simulink model "wamjc7"  (Simulink 8.3)
settings: Solver=ode4  SolverMode=SingleTasking  StartTime=0.0  StopTime=inf  FixedStep=sample_time  RelTol=1e-3
values from neighbouring files (symbols this model uses):
  arm_home = [ -0.1106   -1.9490   -0.1920    3.1840 ]    [NEW_PID_4DOF.m]    (also in SetPoint_Control.m = [ -0.1106   -1.9490   -0.1920    3.1840    0.2825    0.0969 ; Stochastic_coriolis.m = [  -0.1106   -1.9490   -0.1920    3.1840    0.2825    0.0969; Untitled4.m = [ -0.1106   -1.9490   -0.1920    3.1840    0.2825    0.0969 )
  b = 0.001    [DC_motor.m]    (also in SetPoint_Control.m = diag(100*ones(7,1)))
  C = Cjk(q)    [B.m]    (also in DC_motor.m = [1  0  0]; ILC_Grav_Comp.m = [zeros(7,7),eye(7)]; ILC_Grav_Comp_Diff.m = [zeros(7,7),eye(7)]; ILC_Grav_comp_Kalman.m = [zeros(7,7),eye(7)])
undefined symbols (not defined in the file or in its folder): arm_home_norest, arm_j2mt, arm_m2jp, bit, CAN_init, enc_per_rev, FT_init, hand_on, MT_init, puck_I_per_Nm, rotFT2Hand, sample_time, Standard, VL1_init, VL2_init
libraries: xpclib x43, simulink x27, xpcutilitieslib x6, dspmathops x1, dspadpt3 x1, dspindex x1, dspbuff3 x1
(part 1 of 5)
settings Model: xpc_rtwmakecfg_data=_xpccanac2pci_  Creator=Matt Courtney  LastModifiedBy=paulghanem  BufferReuse=off
settings OptimizationCC: BlockReduction=off  BooleanDataType=off  OptimizeBlockIOStorage=off  BufferReuse=off  GlobalBufferReuse=off  ExpressionFolding=off  ExpressionDepthLimit=2147483647  LocalBlockOutputs=off  InitFltsAndDblsToZero=on
settings DebuggingCC: FcnCallInpInsideContextMsg=UseLocalSettings  StrictBusMsg=Warning
settings HardwareCC: ProdIntDivRoundTo=Zero  ProdEndianess=LittleEndian  ProdHWDeviceType=Generic->32-bit x86 compatible
settings SFSimCC: SimParseCustomCode=off
settings RTWCC: SystemTargetFile=xpctarget.tlc  TemplateMakefile=xpc_default_tmf  Description=xPC Target  ProcessScript=xpctarget_make_rtw_hook  RTWCompilerOptimization=On
settings TargetCC: CodeReplacementLibrary=XPC_BLAS  ParMdlRefBuildCompliant=on  ConcurrentExecutionCompliant=on  MatFileLogging=on  EnableShiftOperators=on
settings CustomProperty: DataType=string  Value=Real-Time

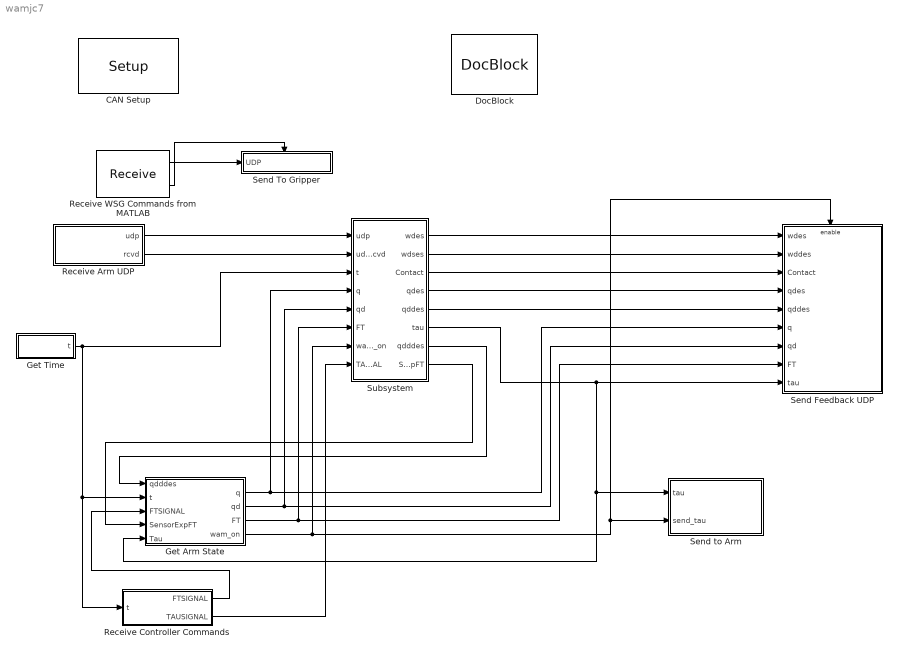
== system wamjc7 ==
  "CAN Setup " : xpclib/CAN/Softing/CAN-AC2-PCI SJA 1000/Setup   board=1  can1bus=Highspeed (ISO 11898)  can1Baudrate=1 MBaud  can1UserBR=[1,1,4,3]  can2bus=Highspeed (ISO 11898)  can2Baudrate=1 MBaud  can2UserBR=[1,1,4,3]  init=[VL1_init,VL2_init,CAN_init,MT_init,FT_init]  term=[]  bus_off_out=off  bus_off_rec=Off  ioBaseAddress=-1
  DocBlock : simulink/Model-Wide Utilities/DocBlock  DocumentType=Text
      content=|
      | This model is a very powerful controller for controlling both the Barrett
      | arm and hand at the same time and in a coordinated fashion. The uppermost
      | block you are looking at contains some CAN initialization commands, as well
      | as the closed loop controllers for the arm and hand. The hand controller
      | is fed the current arm position and velocity every cycle so that it can
      | use this information to intelligently update grasps. Double click the
      | blocks to look at more of the details of each subsystem.
  Get Arm State : Subsystem
  Get Time : Subsystem
  Receive Arm UDP : Subsystem
  Receive Controller Commands : Subsystem
  Receive WSG Commands from MATLAB : xpclib/UDP/Receive  ipAddress=192.168.1.11  ipPort=1500  width=266  vblLen=on  sampletime=sample_time
  Send Feedback UDP : Subsystem
  Send To Gripper : Subsystem  TreatAsAtomicUnit=on
  Send to Arm : Subsystem
  Subsystem : Subsystem
  wires:
  Subsystem/6(tau) -> Send Feedback UDP/9(tau), Send to Arm/1(tau), Get Arm State/5(Tau)
  Get Arm State/1(q) -> Send Feedback UDP/6(q), Subsystem/4(q)
  Get Time/1(t) -> Get Arm State/2(t), Receive Controller Commands/1(t), Subsystem/3(t)
  Subsystem/2(wdses) -> Send Feedback UDP/2(wddes)
  Subsystem/1(wdes) -> Send Feedback UDP/1(wdes)
  Receive Arm UDP/1(udp) -> Subsystem/1(udp)
  Receive Arm UDP/2(rcvd) -> Subsystem/2(udp_rcvd)
  Get Arm State/3(FT) -> Send Feedback UDP/8(FT), Subsystem/6(FT)
  Get Arm State/4(wam_on) -> Send to Arm/2(send_tau), Send Feedback UDP/Enable, Subsystem/7(wam_on)
  Get Arm State/2(qd) -> Send Feedback UDP/7(qd), Subsystem/5(qd)
  Receive Controller Commands/1(FTSIGNAL) -> Get Arm State/3(FTSIGNAL)
  Receive WSG Commands from MATLAB/1 -> Send To Gripper/1(UDP)
  Receive WSG Commands from MATLAB/2 -> Send To Gripper/Trigger
  Subsystem/4(qdes) -> Send Feedback UDP/4(qdes)
  Subsystem/5(qddes) -> Send Feedback UDP/5(qddes)
  Subsystem/7(qdddes) -> Get Arm State/1(qdddes)
  Subsystem/8(SensorExpFT) -> Get Arm State/4(SensorExpFT)
  Subsystem/3(Contact) -> Send Feedback UDP/3(Contact)
  Receive Controller Commands/2(TAUSIGNAL) -> Subsystem/8(TAUSIGNAL)

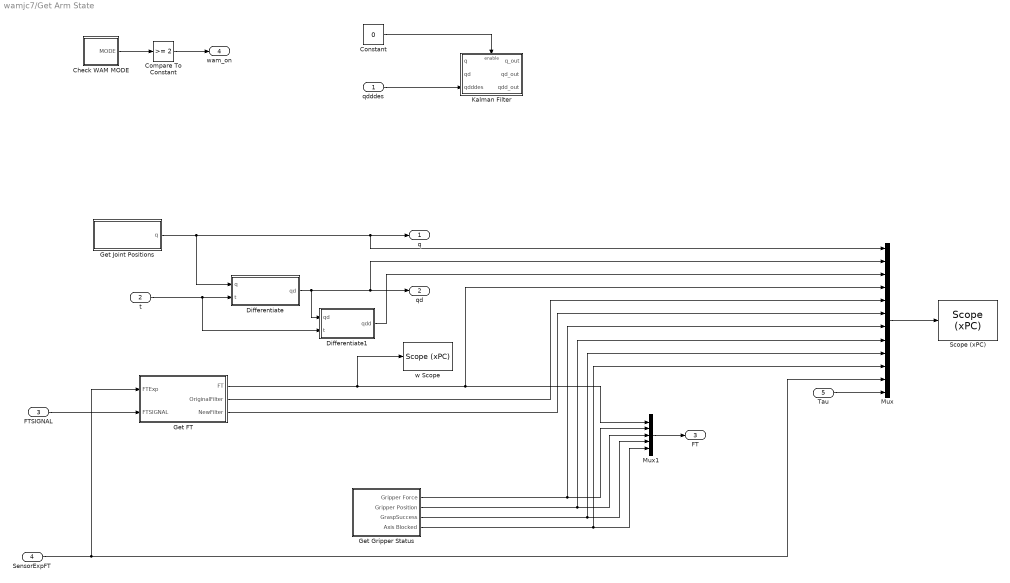
== system wamjc7/Get Arm State ==
  qdddes : Inport
  t : Inport  Port=2
  FTSIGNAL : Inport  Port=3
  SensorExpFT : Inport  Port=4
  Tau : Inport  Port=5
  Check WAM MODE : Subsystem
  Compare To Constant : simulink/Logic and Bit Operations/Compare To Constant  relop=>=  const=2  OutDataTypeStr=uint8  ZeroCross=off
  Constant : Constant  Value=0
  Differentiate : Subsystem
  Differentiate1 : Subsystem
  Get FT : Subsystem
  Get Gripper Status : Subsystem
  Get Joint Positions : Subsystem
  Kalman Filter : Subsystem
  Mux : Mux  Inputs=[7 7 7 6 6 6 1 1 1 1 6 7]
  Mux1 : Mux  Inputs=[6 1 1 1 1]
  "Scope (xPC) " : xpclib/Misc./Scope (xPC)   scopeno=3  scopetype=File  autostart=on  viewmode=Graphical redraw  formatstr='%15.6f'  grid=on  ylimits=[0,0]  nosamples=250  noprepostsamples=0  interleave=1  triggermode=FreeRun  triggersignal=1  triggerlevel=0.0  triggerslope=Either  triggerscope=1  triggersample=0  filename=QFT<%%%>.dat  mode=Lazy  writesize=512  autorestart=on  dynamicfilemode=on  maxwritefilesize=512*1024^2
  w Scope : xpclib/Misc./Scope (xPC)   scopeno=5  scopetype=Target  autostart=on  viewmode=Numerical  formatstr=['Fx %10.5f,Fy %10.5f,Fz %10.5f,TauX %10.5f,TauY %10.5f,TauZ%10.5f']  grid=on  ylimits=[0,0]  nosamples=1/(10*sample_time)  noprepostsamples=0  interleave=1  triggermode=FreeRun  triggersignal=1  triggerlevel=0.0  triggerslope=Either  triggerscope=1  triggersample=0  filename=data.dat  mode=Lazy  writesize=512  autorestart=off  dynamicfilemode=off  maxwritefilesize=512*1024^2
  q : Outport
  qd : Outport  Port=2
  FT : Outport  Port=3
  wam_on : Outport  Port=4
  wires:
  Check WAM MODE/1(MODE) -> Compare To Constant/1
  Differentiate/1(qd) -> Differentiate1/1(qd), qd/1, Mux/2
  Compare To Constant/1 -> wam_on/1
  t/1 -> Differentiate/2(t), Differentiate1/2(t)
  Get Joint Positions/1(q) -> q/1, Mux/1, Differentiate/1(q)
  Mux/1 -> "Scope (xPC) "/1
  Get FT/1(FT) -> w Scope/1, Mux/4, Mux1/1
  FTSIGNAL/1 -> Get FT/2(FTSIGNAL)
  Get FT/2(OriginalFilter) -> Mux/5
  Get FT/3(NewFilter) -> Mux/6
  Differentiate1/1(qdd) -> Mux/3
  Get Gripper Status/1(Gripper Force) -> Mux1/2, Mux/7
  Mux1/1 -> FT/1
  Get Gripper Status/2(Gripper Position) -> Mux1/3, Mux/8
  Get Gripper Status/3(GraspSuccess) -> Mux1/4, Mux/9
  Get Gripper Status/4(Axis Blocked) -> Mux1/5, Mux/10
  Tau/1 -> Mux/12
  Constant/1 -> Kalman Filter/Enable
  qdddes/1 -> Kalman Filter/3(qdddes)
  SensorExpFT/1 -> Get FT/1(FTExp), Mux/11

== system wamjc7/Get Time ==
  Clock Frequency : Constant  Value=1.193e6
  Divide1 : Product  Inputs=*/
  "xPC Target  Time " : xpclib/Misc./xPC Target  Time   ts=sample_time
  t : Outport
  wires:
  "xPC Target  Time "/1 -> Divide1/1
  Clock Frequency/1 -> Divide1/2
  Divide1/1 -> t/1

== system wamjc7/Receive Arm UDP ==
  DocBlock : simulink/Model-Wide Utilities/DocBlock  DocumentType=Text
      content=|
      | We receive UDP trajectory points on port 20202 (for arm). Right now even
      | the gains are sending over UDP but once we find some good gains they should
      | be hard coded in and should not come over UDP. The memory block and logical
      | OR at the bottom is used to check whether or not we have received data
      | since the model started running. If so, we should pass along that data,
      | otherwise we should pass the current position (i.e. the same as being in
      | gravity compensation until some UDP is received)
  Receive : xpclib/UDP/Receive  ipAddress=192.168.1.11  ipPort=5555  width=5992  vblLen=off  sampletime=sample_time
  Unpack : xpclib/UDP/Unpack  dimensions={[749,1]}  datatypes={'double'}  byteAlign=1
  udp : Outport
  rcvd : Outport  Port=2
  wires:
  Unpack/1 -> udp/1
  Receive/1 -> Unpack/1
  Receive/2 -> rcvd/1

== system wamjc7/Receive Controller Commands ==
  t : Inport
  Detect Rise Positive : simulink/Logic and Bit Operations/Detect Rise Positive  vinit=0  InputProcessing=Inherited  OutDataTypeStr=uint8
  DocBlock : simulink/Model-Wide Utilities/DocBlock  DocumentType=Text
  Embedded MATLAB Function : MATLAB Function  TreatAsAtomicUnit=on
  Receive : xpclib/UDP/Receive  ipAddress=192.168.1.11  ipPort=6666  width=9  vblLen=off  sampletime=sample_time
  Unpack : xpclib/UDP/Unpack  dimensions={[9,1]}  datatypes={'uint8'}  byteAlign=1
  FTSIGNAL : Outport
  TAUSIGNAL : Outport  Port=2
  wires:
  Receive/1 -> Unpack/1
  Receive/2 -> Detect Rise Positive/1
  Detect Rise Positive/1 -> Embedded MATLAB Function/3(rcvd)
  Unpack/1 -> Embedded MATLAB Function/2(data)
  t/1 -> Embedded MATLAB Function/1(t)
  Embedded MATLAB Function/1(FTSIGNAL) -> FTSIGNAL/1
  Embedded MATLAB Function/2(TAUSIGNAL) -> TAUSIGNAL/1

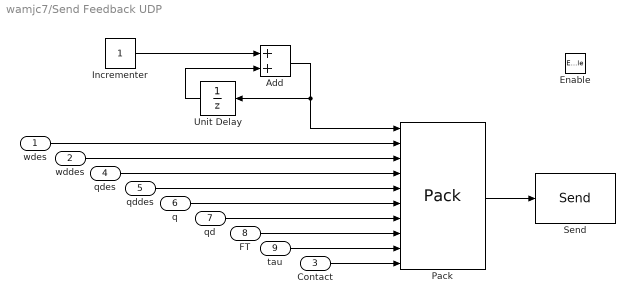
== system wamjc7/Send Feedback UDP ==
  wdes : Inport
  wddes : Inport  Port=2
  Contact : Inport  Port=3
  qdes : Inport  Port=4
  qddes : Inport  Port=5
  q : Inport  Port=6
  qd : Inport  Port=7
  FT : Inport  Port=8
  tau : Inport  Port=9
  Enable : EnablePort  PropagateVarSize=During execution
  Add : Sum  OutDataTypeStr=uint32
  Incrementer : Constant  OutDataTypeStr=uint32
  Pack : xpclib/UDP/Pack  datatypes={'uint32','double','double','double','double','double','double','double','double','double'}  byteAlign=1
  Send : xpclib/UDP/Send  ipAddress=192.168.1.11  ipPort=3333  localPort=-1  vblLen=off  sampletime=sample_time
  Unit Delay : UnitDelay  SampleTime=-1
  wires:
  Pack/1 -> Send/1
  Incrementer/1 -> Add/1
  Unit Delay/1 -> Add/2
  Add/1 -> Pack/1, Unit Delay/1
  qd/1 -> Pack/7
  q/1 -> Pack/6
  qddes/1 -> Pack/5
  qdes/1 -> Pack/4
  wddes/1 -> Pack/3
  wdes/1 -> Pack/2
  tau/1 -> Pack/9
  FT/1 -> Pack/8
  Contact/1 -> Pack/10

== system wamjc7/Send To Gripper ==
  UDP : Inport
  Trigger : TriggerPort
  Send to Gripper : xpclib/UDP/Send  ipAddress=192.168.1.20  ipPort=1500  localPort=-1  vblLen=off  sampletime=-1
  wires:
  UDP/1 -> Send to Gripper/1

== system wamjc7/Send to Arm ==
  tau : Inport
  send_tau : Inport  Port=2
  DocBlock : simulink/Model-Wide Utilities/DocBlock  DocumentType=Text
  Joint Torque to Motor Current : Subsystem
  Pack and Send Torque Packets : Subsystem
  Switch : Switch  Criteria=u2 ~= 0  Threshold=2
  Zero Torques : Constant  Value=[ 0 0 0 0 0 0 0]'  OutDataTypeStr=double
  wires:
  Joint Torque to Motor Current/1(iM) -> Pack and Send Torque Packets/1(Current)
  tau/1 -> Switch/1
  Zero Torques/1 -> Switch/3
  Switch/1 -> Joint Torque to Motor Current/1(tauJ)
  send_tau/1 -> Switch/2

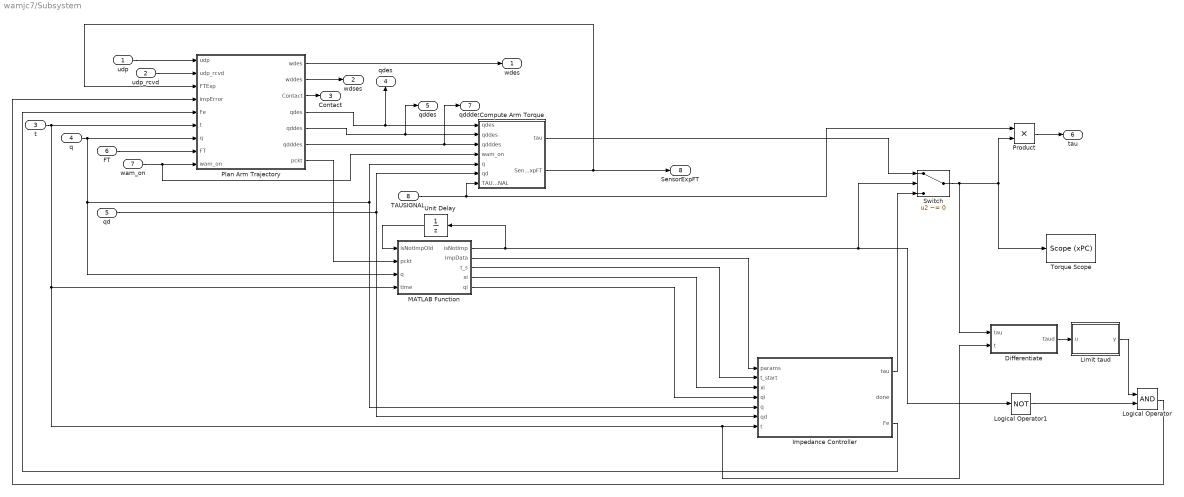
== system wamjc7/Subsystem ==
  udp : Inport
  udp_rcvd : Inport  Port=2
  t : Inport  Port=3
  q : Inport  Port=4
  qd : Inport  Port=5
  FT : Inport  Port=6
  wam_on : Inport  Port=7
  TAUSIGNAL : Inport  Port=8
  Compute Arm Torque : Subsystem
  Differentiate : Subsystem
  Impedance Controller : Subsystem
  Limit taud : MATLAB Function  TreatAsAtomicUnit=on
  Logical Operator : Logic  AllPortsSameDT=off  OutDataTypeStr=boolean
  Logical Operator1 : Logic  Operator=NOT  AllPortsSameDT=off  OutDataTypeStr=boolean
  MATLAB Function : MATLAB Function  TreatAsAtomicUnit=on
  Plan Arm Trajectory : Subsystem
  Product : Product  RndMeth=Zero
  Switch : Switch  Criteria=u2 ~= 0
  Torque Scope : xpclib/Misc./Scope (xPC)   scopeno=10  scopetype=Target  autostart=on  viewmode=Numerical  formatstr=['joint_1 %10.5f N-m,joint_2 %10.5f N-m,joint_3 %10.5f N-m,joint_4 %10.5f N-m,joint_5 %10.5f N-m,joint_6 %10.5f N-m,joint_7 %10.5f N-m']  grid=on  ylimits=[0,0]  nosamples=1/(10*sample_time)  noprepostsamples=0  interleave=1  triggermode=FreeRun  triggersignal=1  triggerlevel=0.0  triggerslope=Either  triggerscope=1  triggersample=0  filename=data.dat  mode=Lazy  writesize=512  autorestart=off  dynamicfilemode=off  maxwritefilesize=512*1024^2
  Unit Delay : UnitDelay  SampleTime=-1
  wdes : Outport
  wdses : Outport  Port=2
  Contact : Outport  Port=3
  qdes : Outport  Port=4
  qddes : Outport  Port=5
  tau : Outport  Port=6
  qdddes : Outport  Port=7
  SensorExpFT : Outport  Port=8
  wires:
  Plan Arm Trajectory/5(qddes) -> qddes/1, Compute Arm Torque/2(qddes)
  Plan Arm Trajectory/6(qdddes) -> Compute Arm Torque/3(qdddes), qdddes/1
  Compute Arm Torque/2(SensorExpFT) -> SensorExpFT/1, Plan Arm Trajectory/3(FTExp)
  t/1 -> Plan Arm Trajectory/6(t), MATLAB Function/4(time), Impedance Controller/7(t), Differentiate/2(t)
  qd/1 -> Compute Arm Torque/6(qd), Impedance Controller/6(qd)
  wam_on/1 -> Plan Arm Trajectory/9(wam_on), Compute Arm Torque/4(wam_on)
  Plan Arm Trajectory/1(wdes) -> wdes/1
  udp/1 -> Plan Arm Trajectory/1(udp)
  udp_rcvd/1 -> Plan Arm Trajectory/2(udp_rcvd)
  Plan Arm Trajectory/2(wddes) -> wdses/1
  Plan Arm Trajectory/3(Contact) -> Contact/1
  FT/1 -> Plan Arm Trajectory/8(FT)
  Unit Delay/1 -> MATLAB Function/1(isNotImpOld)
  MATLAB Function/1(isNotImp) -> Unit Delay/1, Switch/2, Logical Operator1/1
  Plan Arm Trajectory/7(pckt) -> MATLAB Function/2(pckt)
  MATLAB Function/2(ImpData) -> Impedance Controller/1(params)
  MATLAB Function/3(t_s) -> Impedance Controller/2(t_start)
  Impedance Controller/1(tau) -> Switch/3
  Compute Arm Torque/1(tau) -> Switch/1
  Switch/1 -> Differentiate/1(tau), Product/2, Torque Scope/1
  Plan Arm Trajectory/4(qdes) -> Compute Arm Torque/1(qdes), qdes/1
  MATLAB Function/4(xi) -> Impedance Controller/3(xi)
  MATLAB Function/5(qi) -> Impedance Controller/4(qi)
  Differentiate/1(taud) -> Limit taud/1(u)
  Limit taud/1(y) -> Logical Operator/1
  Logical Operator1/1 -> Logical Operator/2
  Logical Operator/1 -> Plan Arm Trajectory/4(impError)
  Impedance Controller/3(Fe) -> Plan Arm Trajectory/5(Fe)
  q/1 -> Plan Arm Trajectory/7(q), MATLAB Function/3(q), Compute Arm Torque/5(q), Impedance Controller/5(q)
  TAUSIGNAL/1 -> Compute Arm Torque/7(TAUSIGNAL), Product/1
  Product/1 -> tau/1

== system wamjc7/Get Arm State/Check WAM MODE ==
  note: Send to lower arm
  "Bit Packing " : xpcutilitieslib/Bit Packing   MaskBitPatterns={[0:7]}  MaskPackDataType=double  MaskPackDataSize=[1]
  Bit Unpacking : xpclib/CAN/Utilities/CAN bit-unpacking   bitpatterns={[16:31]}  dtypes={ 'int16'}
  DocBlock : simulink/Model-Wide Utilities/DocBlock  DocumentType=Text
      content=|
      | Here we send an 8 to the lower arm. Property 8 is the MODE and the
      | 1028 (1 00000 00100) means to "set a lower arm property". Finally we
      | receive the mode property from CAN ID 1158, then do some bit unpacking.
      | All of this is well documentated in the "CAN Communication Spec" of the
      | Barrett documentation.
  Receive lower arm property : xpclib/CAN/Softing/CAN-AC2-PCI SJA 1000/Receive   board=1  canPort=CAN 1  range=Standard (11-bit)  ids=[bin2dec('10010000110')]  lengths=0  output=Data  inten=on  ts=sample_time  ididx=[4]
  Send to all motors 1 : xpclib/CAN/Softing/CAN-AC2-PCI SJA 1000/Send   board=1  canPort=CAN 1  range=Standard (11-bit)  ids=[1028]  sizes=[1]  output=off  ts=sample_time  ididx=[5]
  get MODE : Constant  Value=[8]  OutDataTypeStr=uint8
  MODE : Outport
  wires:
  "Bit Packing "/1 -> Send to all motors 1/1
  Receive lower arm property/1 -> Bit Unpacking/1
  get MODE/1 -> "Bit Packing "/1
  Bit Unpacking/1 -> MODE/1

== system wamjc7/Get Arm State/Differentiate ==
  q : Inport
  t : Inport  Port=2
  Divide : Product  Inputs=*/
  Subtract : Sum  Inputs=+-
  Subtract3 : Sum  Inputs=+-
  Unit Delay : UnitDelay  SampleTime=-1
  Unit Delay1 : UnitDelay  SampleTime=-1
  qd : Outport
  wires:
  q/1 -> Subtract/1, Unit Delay/1
  t/1 -> Unit Delay1/1, Subtract3/1
  Unit Delay1/1 -> Subtract3/2
  Unit Delay/1 -> Subtract/2
  Subtract/1 -> Divide/1
  Divide/1 -> qd/1
  Subtract3/1 -> Divide/2

== system wamjc7/Get Arm State/Differentiate1 ==
  qd : Inport
  t : Inport  Port=2
  Divide : Product  Inputs=*/
  Subtract : Sum  Inputs=+-
  Subtract3 : Sum  Inputs=+-
  Unit Delay : UnitDelay  SampleTime=-1
  Unit Delay1 : UnitDelay  SampleTime=-1
  qdd : Outport
  wires:
  qd/1 -> Subtract/1, Unit Delay/1
  t/1 -> Unit Delay1/1, Subtract3/1
  Unit Delay1/1 -> Subtract3/2
  Unit Delay/1 -> Subtract/2
  Subtract/1 -> Divide/1
  Divide/1 -> qdd/1
  Subtract3/1 -> Divide/2

== system wamjc7/Get Arm State/Get FT ==
  FTExp : Inport
  FTSIGNAL : Inport  Port=2
  Bias FT : Subsystem  TreatAsAtomicUnit=on
  Constant1 : Constant  Value=C  VectorParams1D=off
  Constant2 : Constant  Value=b
  Demux : Demux  Outputs=3
  Get Force Torque : Subsystem
  Matrix Multiply : Product  Multiplication=Matrix(*)
  Sum : Sum  Inputs=+++
  Sum1 : Sum  Inputs=+++
  Sum2 : Sum  Inputs=+++
  Tare FT Sensor : Subsystem  TreatAsAtomicUnit=on
  FT : Outport
  OriginalFilter : Outport  Port=2
  NewFilter : Outport  Port=3
  wires:
  FTSIGNAL/1 -> Demux/1
  Demux/1 -> Tare FT Sensor/Enable, Bias FT/1(RST)
  Demux/3 -> Get Force Torque/Enable
  Demux/2 -> Bias FT/Enable
  Get Force Torque/1(FT) -> Sum/3
  Bias FT/1(Bias) -> Sum/2, Sum2/2, Sum1/2
  Get Force Torque/2(OriginalFilter) -> Sum1/3
  Get Force Torque/3(NewFilter) -> Sum2/3
  Sum2/1 -> NewFilter/1
  Sum1/1 -> OriginalFilter/1
  Constant1/1 -> Matrix Multiply/1
  Matrix Multiply/1 -> FT/1, Bias FT/2(FT)
  Sum/1 -> Matrix Multiply/2
  Constant2/1 -> Sum/1, Sum1/1, Sum2/1
  FTExp/1 -> Bias FT/3(FTExp)

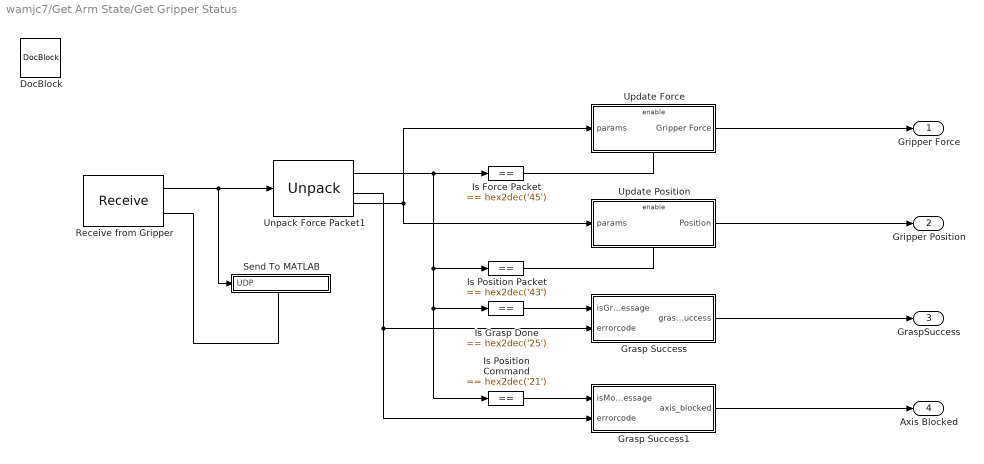
== system wamjc7/Get Arm State/Get Gripper Status ==
  DocBlock : simulink/Model-Wide Utilities/DocBlock  DocumentType=Text
  Grasp Success : MATLAB Function  TreatAsAtomicUnit=on
  Grasp Success1 : MATLAB Function  TreatAsAtomicUnit=on
  Is Force Packet : simulink/Logic and Bit Operations/Compare To Constant  relop===  const=hex2dec('45')  OutDataTypeStr=uint8
  Is Grasp Done : simulink/Logic and Bit Operations/Compare To Constant  relop===  const=hex2dec('25')  OutDataTypeStr=uint8
  Is Position Command : simulink/Logic and Bit Operations/Compare To Constant  relop===  const=hex2dec('21')  OutDataTypeStr=uint8
  Is Position Packet : simulink/Logic and Bit Operations/Compare To Constant  relop===  const=hex2dec('43')  OutDataTypeStr=uint8
  Receive from Gripper : xpclib/UDP/Receive  ipAddress=192.168.1.20  ipPort=1501  width=266  vblLen=on  sampletime=sample_time
  Send To MATLAB : Subsystem  TreatAsAtomicUnit=on
  Unpack Force Packet1 : xpclib/UDP/Unpack  dimensions={3,1,1,1,1,254}  datatypes={'uint8','uint8','uint16','uint16','single','uint8'}  byteAlign=1
  Update Force : Subsystem  TreatAsAtomicUnit=on
  Update Position : Subsystem  TreatAsAtomicUnit=on
  Gripper Force : Outport
  Gripper Position : Outport  Port=2
  GraspSuccess : Outport  Port=3
  Axis Blocked : Outport  Port=4
  wires:
  Receive from Gripper/2 -> Send To MATLAB/Trigger
  Receive from Gripper/1 -> Send To MATLAB/1(UDP), Unpack Force Packet1/1
  Unpack Force Packet1/5 -> Update Force/1(params), Update Position/1(params)
  Unpack Force Packet1/2 -> Is Force Packet/1, Is Position Packet/1, Is Grasp Done/1, Is Position Command/1
  Update Force/1(Gripper Force) -> Gripper Force/1
  Is Force Packet/1 -> Update Force/Enable
  Is Position Packet/1 -> Update Position/Enable
  Update Position/1(Position) -> Gripper Position/1
  Unpack Force Packet1/4 -> Grasp Success/2(errorcode), Grasp Success1/2(errorcode)
  Is Grasp Done/1 -> Grasp Success/1(isGraspMessage)
  Grasp Success/1(grasp_success) -> GraspSuccess/1
  Grasp Success1/1(axis_blocked) -> Axis Blocked/1
  Is Position Command/1 -> Grasp Success1/1(isMoveFingerMessage)

== system wamjc7/Get Arm State/Get Joint Positions ==
  DocBlock : simulink/Model-Wide Utilities/DocBlock  DocumentType=Text
  Filter Bad Readings : Subsystem
  Motor Counts to Joint Radians : Subsystem
  Recieve and Unpack  Motor Positions : Subsystem
  Send Get Position : Subsystem
  q : Outport
  wires:
  Recieve and Unpack  Motor Positions/1(qM) -> Filter Bad Readings/1(qM_in)
  Motor Counts to Joint Radians/1(qJ) -> q/1
  Filter Bad Readings/1(qM_out) -> Motor Counts to Joint Radians/1(qM)

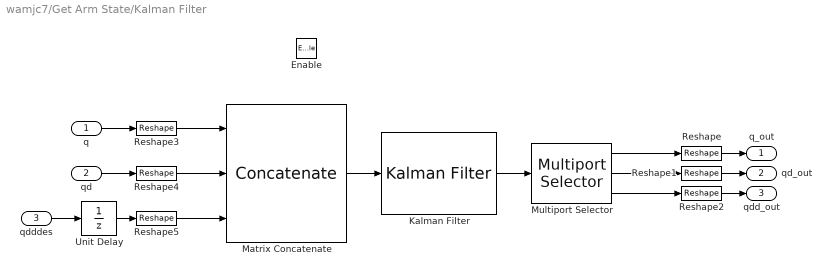
== system wamjc7/Get Arm State/Kalman Filter ==
  q : Inport
  qd : Inport  Port=2
  qdddes : Inport  Port=3
  Enable : EnablePort
  Kalman Filter : dspadpt3/Kalman Filter  num_targets=7  sourceEnable=Always  isReset=on  X=[0 0 0 0 0]'  P=10*eye(5)  A=[1 sample_time 0 0 0 ;0 1 sample_time 0 0; 0 0 1 sample_time 0; 0 0 0 1 sample_time; 0 0 0 0 1]  sourceMeasure=Specify via Dialog  H=[1 0 0 0 0; 0 1 0 0 0; 0 0 1 0 0]  Q=diag([1e-6 1e-6 1e-6 1e-6 1e-0])*eye(5)  R=diag([1e-4 0.5 1.0])*eye(3)  isOutputEstMeasure=off  isOutputEstState=on  isOutputEstError=off  isOutputPrdMeasure=off  isOutputPrdState=off  isOutputPrdError=off
  Matrix Concatenate : Concatenate  NumInputs=3  Mode=Multidimensional array
  Multiport Selector : dspindex/Multiport Selector  rowsOrCols=Rows  idxCellArray={ 1,2,3}  idxErrMode=Clip Index
  Reshape : Reshape
  Reshape1 : Reshape
  Reshape2 : Reshape
  Reshape3 : Reshape  OutputDimensionality=Customize  OutputDimensions=[1,7]
  Reshape4 : Reshape  OutputDimensionality=Customize  OutputDimensions=[1,7]
  Reshape5 : Reshape  OutputDimensionality=Customize  OutputDimensions=[1,7]
  Unit Delay : UnitDelay  SampleTime=-1
  q_out : Outport
  qd_out : Outport  Port=2
  qdd_out : Outport  Port=3
  wires:
  Matrix Concatenate/1 -> Kalman Filter/1
  Kalman Filter/1 -> Multiport Selector/1
  Multiport Selector/1 -> Reshape/1
  Multiport Selector/2 -> Reshape1/1
  Multiport Selector/3 -> Reshape2/1
  Reshape5/1 -> Matrix Concatenate/3
  Reshape3/1 -> Matrix Concatenate/1
  Reshape4/1 -> Matrix Concatenate/2
  Unit Delay/1 -> Reshape5/1
  qdddes/1 -> Unit Delay/1
  q/1 -> Reshape3/1
  qd/1 -> Reshape4/1
  Reshape/1 -> q_out/1
  Reshape1/1 -> qd_out/1
  Reshape2/1 -> qdd_out/1

== system wamjc7/Send to Arm/Joint Torque to Motor Current ==
  tauJ : Inport
  DocBlock : simulink/Model-Wide Utilities/DocBlock  DocumentType=Text
  J2M Torque Matrix : Constant  Value=arm_j2mt
  Matrix Multiply : Product  Multiplication=Matrix(*)
  Product : Product  RndMeth=Zero
  puckIperNm : Constant  Value=puck_I_per_Nm
  iM : Outport
  wires:
  J2M Torque Matrix/1 -> Matrix Multiply/1
  Matrix Multiply/1 -> Product/2
  puckIperNm/1 -> Product/1
  Product/1 -> iM/1
  tauJ/1 -> Matrix Multiply/2

== system wamjc7/Send to Arm/Pack and Send Torque Packets ==
  Current : Inport
  Bit Packing : xpcutilitieslib/Bit Packing   MaskBitPatterns={[0:7] [18:23 8:15] [36:39 24:31 16:17] [54:55 40:47 32:35] [56:63 48:53]}  MaskPackDataType=double  MaskPackDataSize=[1]
  Bit Packing1 : xpcutilitieslib/Bit Packing   MaskBitPatterns={[0:7] [18:23 8:15] [36:39 24:31 16:17] [54:55 40:47 32:35] [56:63 48:53]}  MaskPackDataType=double  MaskPackDataSize=[1]
  Data Type Conversion1 : DataTypeConversion  OutMin=[-8191]  OutMax=[8191]  OutDataTypeStr=int16  RndMeth=Zero
  Demux2 : Demux  Outputs=7
  DocBlock : simulink/Model-Wide Utilities/DocBlock  DocumentType=Text
  Send to Lower Arm : xpclib/CAN/Softing/CAN-AC2-PCI SJA 1000/Send   board=1  canPort=CAN 1  range=Standard (11-bit)  ids=bin2dec('10000000001')  sizes=[8]  output=off  ts=sample_time  ididx=[3]
  Send to Upper Arm : xpclib/CAN/Softing/CAN-AC2-PCI SJA 1000/Send   board=1  canPort=CAN 1  range=Standard (11-bit)  ids=bin2dec('10000000010')  sizes=[8]  output=off  ts=sample_time  ididx=[4]
  "Set Torques " : Constant  Value=[170]  OutDataTypeStr=uint8
  Zero : Constant  Value=0  OutDataTypeStr=int16
  wires:
  "Set Torques "/1 -> Bit Packing/1, Bit Packing1/1
  Bit Packing/1 -> Send to Lower Arm/1
  Demux2/1 -> Bit Packing/2
  Demux2/2 -> Bit Packing/3
  Demux2/3 -> Bit Packing/4
  Demux2/4 -> Bit Packing/5
  Current/1 -> Data Type Conversion1/1
  Data Type Conversion1/1 -> Demux2/1
  Bit Packing1/1 -> Send to Upper Arm/1
  Demux2/5 -> Bit Packing1/2
  Demux2/6 -> Bit Packing1/3
  Demux2/7 -> Bit Packing1/4
  Zero/1 -> Bit Packing1/5

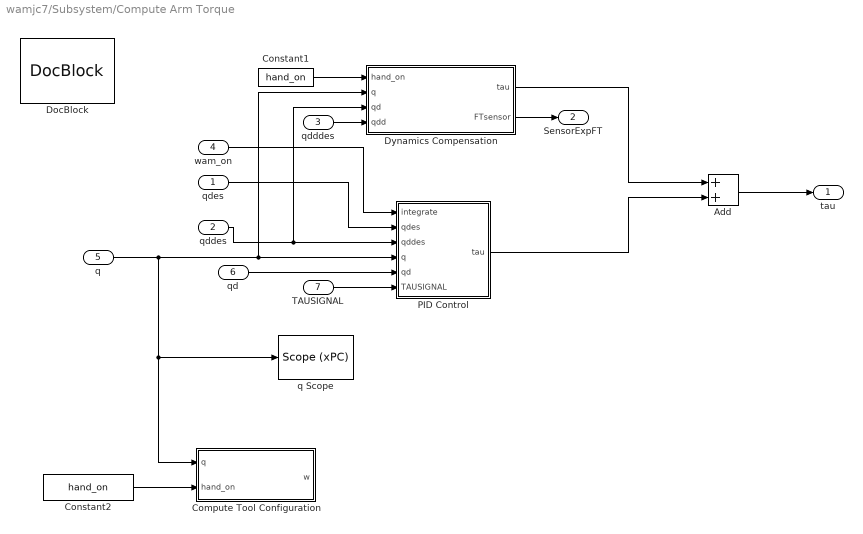
== system wamjc7/Subsystem/Compute Arm Torque ==
  qdes : Inport
  qddes : Inport  Port=2
  qdddes : Inport  Port=3
  wam_on : Inport  Port=4
  q : Inport  Port=5
  qd : Inport  Port=6
  TAUSIGNAL : Inport  Port=7
  Add : Sum
  Compute Tool Configuration : MATLAB Function  TreatAsAtomicUnit=on
  Constant1 : Constant  Value=hand_on
  Constant2 : Constant  Value=hand_on
  DocBlock : simulink/Model-Wide Utilities/DocBlock  DocumentType=Text
      content=|
      | This is where the control happens. We take the current position and
      | velocity as input, and pass those to a PID block which then pushes out a
      | desired acceleration. The desired accelerations go through Recursive Newton
      | Euler which then outputs the appropriate torques to be sent to the WAM
  Dynamics Compensation : MATLAB Function  TreatAsAtomicUnit=on
  PID Control : Subsystem
  q Scope : xpclib/Misc./Scope (xPC)   scopeno=9  scopetype=Target  autostart=on  viewmode=Numerical  formatstr=['joint_1 %10.5f rad,joint_2 %10.5f rad,joint_3 %10.5f rad,joint_4 %10.5f rad,joint_5 %10.5f rad,joint_6 %10.5f rad,joint_7 %10.5f rad']  grid=on  ylimits=[0,0]  nosamples=1/(10*sample_time)  noprepostsamples=0  interleave=1  triggermode=FreeRun  triggersignal=1  triggerlevel=0.0  triggerslope=Either  triggerscope=1  triggersample=0  filename=data.dat  mode=Lazy  writesize=512  autorestart=off  dynamicfilemode=off  maxwritefilesize=512*1024^2
  tau : Outport
  SensorExpFT : Outport  Port=2
  wires:
  qd/1 -> PID Control/5(qd)
  Add/1 -> tau/1
  q/1 -> PID Control/4(q), Dynamics Compensation/2(q), Compute Tool Configuration/1(q), q Scope/1
  wam_on/1 -> PID Control/1(integrate)
  qddes/1 -> PID Control/3(qddes), Dynamics Compensation/3(qd)
  qdes/1 -> PID Control/2(qdes)
  PID Control/1(tau) -> Add/2
  Constant2/1 -> Compute Tool Configuration/2(hand_on)
  Dynamics Compensation/1(tau) -> Add/1
  Constant1/1 -> Dynamics Compensation/1(hand_on)
  qdddes/1 -> Dynamics Compensation/4(qdd)
  Dynamics Compensation/2(FTsensor) -> SensorExpFT/1
  TAUSIGNAL/1 -> PID Control/6(TAUSIGNAL)

== system wamjc7/Subsystem/Differentiate ==
  tau : Inport
  t : Inport  Port=2
  Divide : Product  Inputs=*/
  Subtract : Sum  Inputs=+-
  Subtract3 : Sum  Inputs=+-
  Unit Delay : UnitDelay  SampleTime=-1
  Unit Delay1 : UnitDelay  SampleTime=-1
  taud : Outport
  wires:
  tau/1 -> Subtract/1, Unit Delay/1
  t/1 -> Unit Delay1/1, Subtract3/1
  Unit Delay1/1 -> Subtract3/2
  Unit Delay/1 -> Subtract/2
  Subtract/1 -> Divide/1
  Divide/1 -> taud/1
  Subtract3/1 -> Divide/2

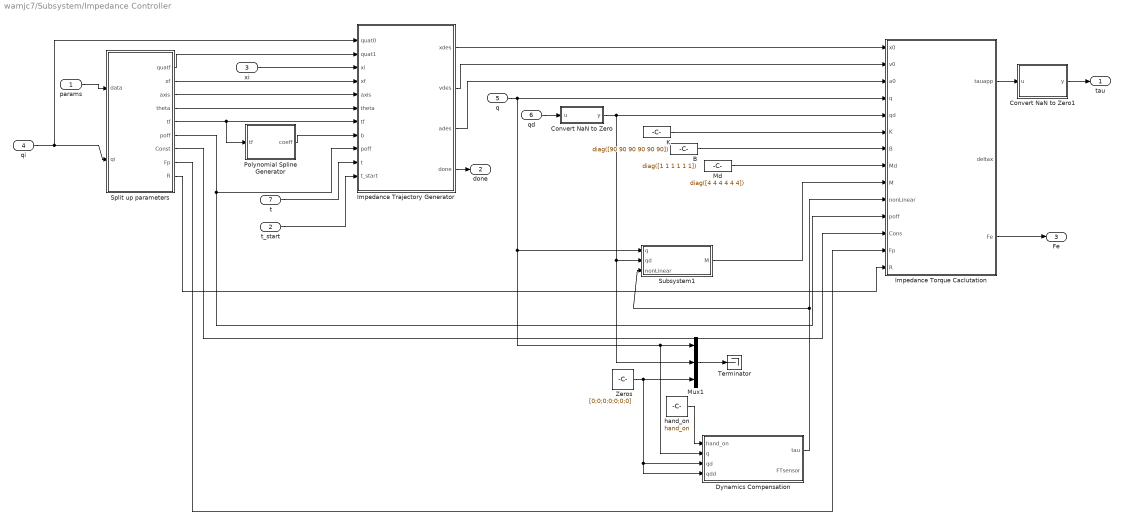
== system wamjc7/Subsystem/Impedance Controller ==
  params : Inport
  t_start : Inport  Port=2
  xi : Inport  Port=3
  qi : Inport  Port=4
  q : Inport  Port=5
  qd : Inport  Port=6
  t : Inport  Port=7
  B : Constant  Value=diag([1 1 1 1 1 1])  VectorParams1D=off
  Convert NaN to Zero : MATLAB Function  TreatAsAtomicUnit=on
  Convert NaN to Zero1 : MATLAB Function  TreatAsAtomicUnit=on
  Dynamics Compensation : MATLAB Function  TreatAsAtomicUnit=on
  Impedance Torque Caclutation : MATLAB Function  TreatAsAtomicUnit=on
  Impedance Trajectory Generator : MATLAB Function  TreatAsAtomicUnit=on
  K : Constant  Value=diag([90 90 90 90 90 90])  VectorParams1D=off
  Md : Constant  Value=diag([4 4 4 4 4 4])  VectorParams1D=off
  Mux1 : Mux  Inputs=3
  Polynomial Spline Generator : MATLAB Function  TreatAsAtomicUnit=on
  Split up parameters : MATLAB Function  TreatAsAtomicUnit=on
  Subsystem1 : Subsystem
  Terminator : Terminator
  Zeros : Constant  Value=[0;0;0;0;0;0;0]
  hand_on : Constant  Value=hand_on
  tau : Outport
  done : Outport  Port=2
  Fe : Outport  Port=3
  wires:
  params/1 -> Split up parameters/1(data)
  Zeros/1 -> Mux1/3, Dynamics Compensation/4(qdd), Dynamics Compensation/3(qd)
  Dynamics Compensation/1(tau) -> Impedance Torque Caclutation/10(nonLinear), Subsystem1/3(nonLinear)
  Split up parameters/5(tf) -> Polynomial Spline Generator/1(tf), Impedance Trajectory Generator/7(tf)
  Polynomial Spline Generator/1(coeff) -> Impedance Trajectory Generator/8(b)
  Split up parameters/4(theta) -> Impedance Trajectory Generator/6(theta)
  Split up parameters/1(quatf) -> Impedance Trajectory Generator/2(quat1)
  Impedance Trajectory Generator/1(xdes) -> Impedance Torque Caclutation/1(x0)
  Impedance Trajectory Generator/2(vdes) -> Impedance Torque Caclutation/2(v0)
  Impedance Trajectory Generator/3(ades) -> Impedance Torque Caclutation/3(a0)
  q/1 -> Impedance Torque Caclutation/4(q), Subsystem1/1(q), Mux1/1, Dynamics Compensation/2(q)
  t/1 -> Impedance Trajectory Generator/10(t)
  K/1 -> Impedance Torque Caclutation/6(K)
  B/1 -> Impedance Torque Caclutation/7(B)
  Md/1 -> Impedance Torque Caclutation/8(Md)
  t_start/1 -> Impedance Trajectory Generator/11(t_start)
  qd/1 -> Convert NaN to Zero/1(u)
  Convert NaN to Zero/1(y) -> Impedance Torque Caclutation/5(qd), Subsystem1/2(qd), Mux1/2
  Subsystem1/1(M) -> Impedance Torque Caclutation/9(M)
  hand_on/1 -> Dynamics Compensation/1(hand_on)
  xi/1 -> Impedance Trajectory Generator/3(xi)
  Split up parameters/6(poff) -> Impedance Torque Caclutation/11(poff), Impedance Trajectory Generator/9(poff)
  Split up parameters/7(Const) -> Impedance Torque Caclutation/12(Cons)
  Split up parameters/8(Fp) -> Impedance Torque Caclutation/13(Fp)
  Impedance Torque Caclutation/3(Fe) -> Fe/1
  Impedance Torque Caclutation/1(tauapp) -> Convert NaN to Zero1/1(u)
  Convert NaN to Zero1/1(y) -> tau/1
  Impedance Trajectory Generator/4(done) -> done/1
  Mux1/1 -> Terminator/1
  qi/1 -> Split up parameters/2(qi), Impedance Trajectory Generator/1(quat0)
  Split up parameters/2(xf) -> Impedance Trajectory Generator/4(xf)
  Split up parameters/3(axis) -> Impedance Trajectory Generator/5(axis)
  Split up parameters/9(R) -> Impedance Torque Caclutation/14(R)

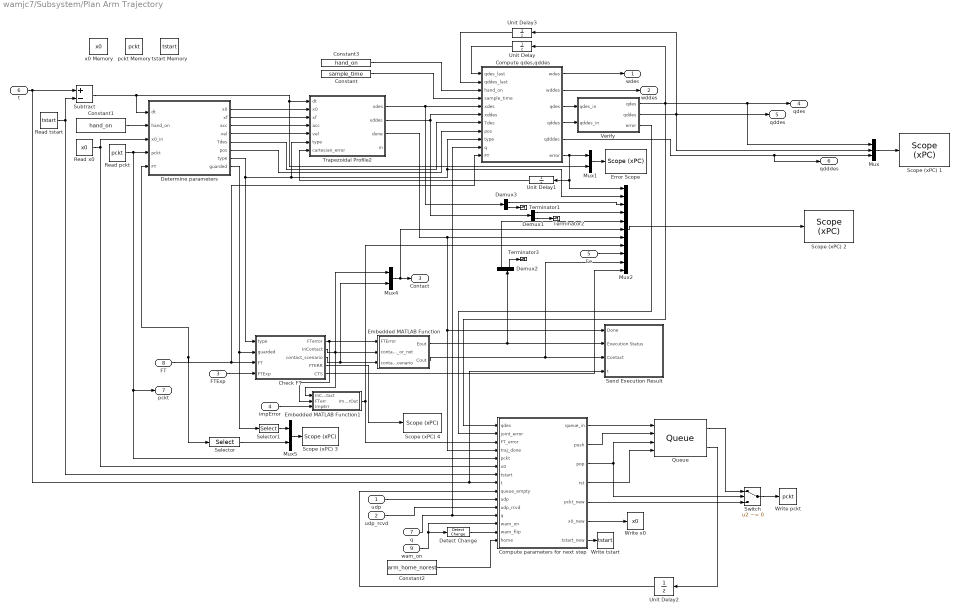
== system wamjc7/Subsystem/Plan Arm Trajectory ==
  udp : Inport
  udp_rcvd : Inport  Port=2
  FTExp : Inport  Port=3
  impError : Inport  Port=4
  Fe : Inport  Port=5
  t : Inport  Port=6
  q : Inport  Port=7
  FT : Inport  Port=8
  wam_on : Inport  Port=9
  Check FT : MATLAB Function  TreatAsAtomicUnit=on
  Compute parameters for next step : MATLAB Function  TreatAsAtomicUnit=on
  Compute qdes,qddes : MATLAB Function  TreatAsAtomicUnit=on
  Constant : Constant  Value=sample_time
  Constant1 : Constant  Value=hand_on
  Constant2 : Constant  Value=arm_home_norest
  Constant3 : Constant  Value=hand_on
  Demux1 : Demux  Outputs=[3 4]
  Demux2 : Demux  Outputs=[1 2]
  Demux3 : Demux  Outputs=[3 4]
  Detect Change : simulink/Logic and Bit Operations/Detect Change  vinit=0  InputProcessing=Inherited  OutDataTypeStr=uint8
  Determine parameters : MATLAB Function  TreatAsAtomicUnit=on
  Embedded MATLAB Function : MATLAB Function  TreatAsAtomicUnit=on
  Embedded MATLAB Function1 : MATLAB Function  TreatAsAtomicUnit=on
  Error Scope : xpclib/Misc./Scope (xPC)   scopeno=1  scopetype=Target  autostart=on  viewmode=Numerical  formatstr=['x_err %10.5f m,y_err %10.5f m,z_err %10.5f m,rx_err %10.5f,ry_err %10.5f,rz_err %10.5f,dt %10.5f']  grid=on  ylimits=[0,0]  nosamples=1/(10*sample_time)  noprepostsamples=0  interleave=1  triggermode=FreeRun  triggersignal=1  triggerlevel=0.0  triggerslope=Either  triggerscope=1  triggersample=0  filename=data.dat  mode=Lazy  writesize=512  autorestart=off  dynamicfilemode=off  maxwritefilesize=512*1024^2
  Mux : Mux  Inputs=[7 7 7]
  Mux1 : Mux  Inputs=[6 1]
  Mux2 : Mux  Inputs=[6 1 3 3 1 2 1 1 6 2 2]
  Mux4 : Mux  Inputs=[1 1]
  Mux5 : Mux  Inputs=[4 2]
  Queue : dspbuff3/Queue  depth=1  trigger=Non-zero sample  overflow=Ignore  pes=Warning  eso=on  fso=off  nso=off  clr=on  clrOutport=off  adf=on
  Read pckt : DataStoreRead  DataStoreName=pckt
  Read tstart : DataStoreRead  DataStoreName=tstart
  Read x0 : DataStoreRead  DataStoreName=x0
  Scope (xPC) 1 : xpclib/Misc./Scope (xPC)   scopeno=2  scopetype=File  autostart=on  viewmode=Graphical redraw  formatstr='%15.6f'  grid=on  ylimits=[0,0]  nosamples=250  noprepostsamples=0  interleave=1  triggermode=FreeRun  triggersignal=1  triggerlevel=0.0  triggerslope=Either  triggerscope=1  triggersample=0  filename=Qdes<%%%>.dat  mode=Lazy  writesize=512  autorestart=on  dynamicfilemode=on  maxwritefilesize=512*1024^2
  Scope (xPC) 2 : xpclib/Misc./Scope (xPC)   scopeno=4  scopetype=File  autostart=on  viewmode=Graphical redraw  formatstr='%15.6f'  grid=on  ylimits=[0,0]  nosamples=250  noprepostsamples=0  interleave=1  triggermode=FreeRun  triggersignal=1  triggerlevel=0.0  triggerslope=Either  triggerscope=1  triggersample=0  filename=ERROR<%%%>.dat  mode=Lazy  writesize=512  autorestart=on  dynamicfilemode=on  maxwritefilesize=512*1024^2
  Scope (xPC) 3 : xpclib/Misc./Scope (xPC)   scopeno=6  scopetype=Target  autostart=on  viewmode=Numerical  formatstr='Guard %15.6f,STime %15.6f,AdjType %15.6f,Squeeze %15.6,GripF %15.6f,GripW %15.6f'  grid=on  ylimits=[0,0]  nosamples=250  noprepostsamples=0  interleave=1  triggermode=FreeRun  triggersignal=1  triggerlevel=0.0  triggerslope=Either  triggerscope=1  triggersample=0  filename=ERROR<%%%>1.dat  mode=Lazy  writesize=512  autorestart=on  dynamicfilemode=on  maxwritefilesize=512*1024^2
  Scope (xPC) 4 : xpclib/Misc./Scope (xPC)   scopeno=7  scopetype=Target  autostart=on  viewmode=Numerical  formatstr='%15.6f'  grid=on  ylimits=[0,0]  nosamples=250  noprepostsamples=0  interleave=1  triggermode=FreeRun  triggersignal=1  triggerlevel=0.0  triggerslope=Either  triggerscope=1  triggersample=0  filename=ERROR<%%%>1.dat  mode=Lazy  writesize=512  autorestart=on  dynamicfilemode=on  maxwritefilesize=512*1024^2
  Selector : Selector  InputPortWidth=10  Indices=[7,8]
  Selector1 : Selector  InputPortWidth=5  Indices=[1,2,4,5]
  Send Execution Result : Subsystem  TreatAsAtomicUnit=on
  Subtract : Sum  Inputs=+-
  Switch : Switch  Criteria=u2 ~= 0
  Terminator1 : Terminator
  Terminator2 : Terminator
  Terminator3 : Terminator
  Trapezoidal Profile2 : MATLAB Function  TreatAsAtomicUnit=on
  Unit Delay : UnitDelay  SampleTime=-1
  Unit Delay1 : UnitDelay  InitialCondition=1  SampleTime=-1
  Unit Delay2 : UnitDelay  InitialCondition=1  SampleTime=-1
  Unit Delay3 : UnitDelay  SampleTime=-1
  Verify : MATLAB Function  TreatAsAtomicUnit=on
  Write pckt : DataStoreWrite  DataStoreName=pckt
  Write tstart : DataStoreWrite  DataStoreName=tstart
  Write x0 : DataStoreWrite  DataStoreName=x0
  pckt Memory : DataStoreMemory  DataStoreName=pckt  InitialValue=[0 0 pi/4 0 pi/2 0 0.1 0 zeros(1,741)]'
  tstart Memory : DataStoreMemory  DataStoreName=tstart
  x0 Memory : DataStoreMemory  DataStoreName=x0  InitialValue=arm_home'
  wdes : Outport
  wddes : Outport  Port=2
  Contact : Outport  Port=3
  qdes : Outport  Port=4
  qddes : Outport  Port=5
  qdddes : Outport  Port=6
  pckt : Outport  Port=7
  wires:
  t/1 -> Subtract/1, Compute parameters for next step/8(t), Send Execution Result/4(t)
  Read tstart/1 -> Subtract/2, Compute parameters for next step/7(tstart)
  Read x0/1 -> Compute parameters for next step/6(x0), Determine parameters/3(x0_in)
  Read pckt/1 -> Determine parameters/4(pckt), Compute parameters for next step/5(pckt), pckt/1
  Compute parameters for next step/7(tstart_new) -> Write tstart/1
  Compute parameters for next step/6(x0_new) -> Write x0/1
  wam_on/1 -> Compute parameters for next step/13(wam_on), Detect Change/1
  Queue/2 -> Unit Delay2/1
  q/1 -> Compute parameters for next step/12(q), Compute qdes,qddes/10(q)
  Compute parameters for next step/3(pop) -> Queue/3, Switch/2
  Compute parameters for next step/4(rst) -> Queue/4
  Unit Delay2/1 -> Compute parameters for next step/9(queue_empty)
  Compute parameters for next step/2(push) -> Queue/2
  Compute parameters for next step/1(queue_in) -> Queue/1
  udp_rcvd/1 -> Compute parameters for next step/11(udp_rcvd)
  udp/1 -> Compute parameters for next step/10(udp)
  Constant1/1 -> Determine parameters/2(hand_on)
  Queue/1 -> Switch/1
  Compute parameters for next step/5(pckt_new) -> Switch/3
  Switch/1 -> Write pckt/1
  Detect Change/1 -> Compute parameters for next step/14(wam_flip)
  Constant2/1 -> Compute parameters for next step/15(home)
  Unit Delay/1 -> Compute qdes,qddes/1(qdes_last)
  Constant/1 -> Compute qdes,qddes/4(sample_time)
  Subtract/1 -> Trapezoidal Profile2/1(dt), Mux1/2, Determine parameters/1(dt)
  Determine parameters/1(x0) -> Trapezoidal Profile2/2(x0)
  Determine parameters/2(xf) -> Trapezoidal Profile2/3(xf)
  Determine parameters/3(acc) -> Trapezoidal Profile2/4(acc)
  Determine parameters/4(vel) -> Trapezoidal Profile2/5(vel)
  Determine parameters/6(pos) -> Compute qdes,qddes/8(pos)
  Constant3/1 -> Compute qdes,qddes/3(hand_on)
  Compute qdes,qddes/1(wdes) -> wdes/1
  Compute qdes,qddes/2(wddes) -> wddes/1
  Determine parameters/5(Tdes) -> Compute qdes,qddes/7(Tdes)
  Trapezoidal Profile2/1(xdes) -> Compute qdes,qddes/5(xdes), Demux3/1
  Trapezoidal Profile2/2(xddes) -> Compute qdes,qddes/6(xddes), Demux1/1
  Compute qdes,qddes/3(qdes) -> Verify/1(qdes_in)
  Compute qdes,qddes/4(qddes) -> Verify/2(qddes_in)
  Verify/3(error) -> Compute parameters for next step/2(joint_error)
  Compute qdes,qddes/6(error) -> Mux1/1, Unit Delay1/1, Mux2/1
  Unit Delay1/1 -> Trapezoidal Profile2/7(cartesian_error)
  Verify/2(qddes) -> Unit Delay3/1, Mux/2, qddes/1
  Verify/1(qdes) -> Unit Delay/1, Compute parameters for next step/1(qdes), qdes/1, Mux/1
  Mux/1 -> Scope (xPC) 1/1
  Mux1/1 -> Error Scope/1
  Determine parameters/7(type) -> Trapezoidal Profile2/6(type), Compute qdes,qddes/9(type), Mux2/2, Check FT/1(type)
  Demux1/1 -> Mux2/4
  Unit Delay3/1 -> Compute qdes,qddes/2(qddes_last)
  Compute qdes,qddes/5(qdddes) -> Mux/3, qdddes/1
  FT/1 -> Determine parameters/5(FT), Selector/1, Check FT/3(FT), Compute qdes,qddes/11(FT)
  FTExp/1 -> Check FT/4(FTExp)
  Check FT/4(FTERR) -> Scope (xPC) 4/1
  Check FT/2(InContact) -> Embedded MATLAB Function1/1(InContact), Mux4/1, Embedded MATLAB Function/2(contact_or_not)
  Check FT/3(contact_scenario) -> Mux4/2, Embedded MATLAB Function/3(contact_scenario)
  Mux4/1 -> Contact/1, Mux2/6
  Mux5/1 -> Scope (xPC) 3/1
  Selector/1 -> Mux5/2
  Selector1/1 -> Mux5/1
  Embedded MATLAB Function/1(Eout) -> Demux2/1, Send Execution Result/2(Execution Status)
  Embedded MATLAB Function/2(Cout) -> Send Execution Result/3(Contact), Mux2/10
  Demux2/2 -> Terminator3/1
  Demux1/2 -> Terminator2/1
  Demux3/2 -> Terminator1/1
  Determine parameters/8(guarded) -> Selector1/1, Check FT/2(guarded)
  Trapezoidal Profile2/3(done) -> Compute parameters for next step/4(traj_done), Send Execution Result/1(Done), Mux2/7
  Demux2/1 -> Mux2/5
  impError/1 -> Embedded MATLAB Function1/3(ImpErr)
  Check FT/1(FTerror) -> Embedded MATLAB Function1/2(FTerr), Embedded MATLAB Function/1(FTError)
  Fe/1 -> Mux2/9
  Mux2/1 -> Scope (xPC) 2/1
  Demux3/1 -> Mux2/3
  Embedded MATLAB Function1/1(ImpErrOut) -> Mux2/8, Compute parameters for next step/3(FT_error)
  Check FT/5(CTS) -> Mux2/11

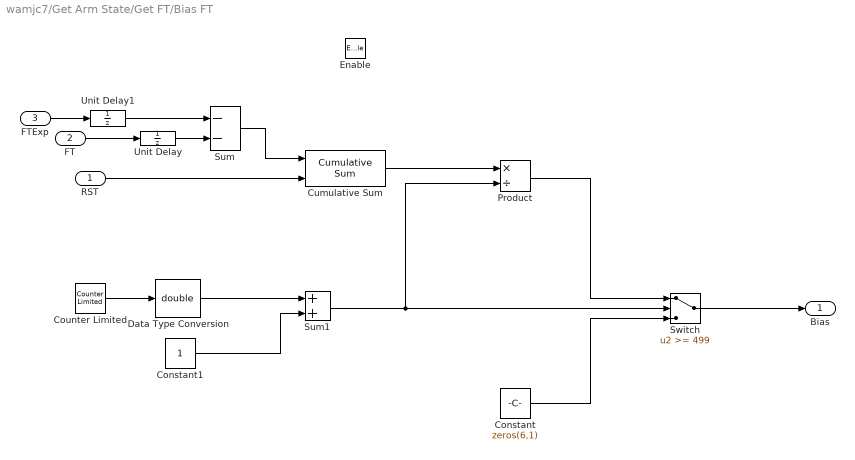
== system wamjc7/Get Arm State/Get FT/Bias FT ==
  RST : Inport
  FT : Inport  Port=2
  FTExp : Inport  Port=3
  Enable : EnablePort  StatesWhenEnabling=reset
  Constant : Constant  Value=zeros(6,1)
  Constant1 : Constant
  Counter Limited : simulink/Sources/Counter Limited  uplimit=500  tsamp=-1
  Cumulative Sum : dspmathops/Cumulative Sum  dim=Channels (running sum)  InputProcessing=Inherited (this choice will be removed - see release notes)  reset_popup=Non-zero sample  outputDataTypeStr=Inherit: Same as accumulator  outputLastDataTypeStr=Inherit: Same as accumulator  outputMin=[]  outputMax=[]  roundingMode=Floor  overflowMode=off
  Data Type Conversion : DataTypeConversion  OutDataTypeStr=double
  Product : Product  Inputs=*/  RndMeth=Zero
  Sum : Sum  Inputs=--
  Sum1 : Sum
  Switch : Switch  Threshold=499
  Unit Delay : UnitDelay  SampleTime=-1
  Unit Delay1 : UnitDelay  SampleTime=-1
  Bias : Outport
  wires:
  RST/1 -> Cumulative Sum/2
  Cumulative Sum/1 -> Product/1
  Product/1 -> Switch/1
  Counter Limited/1 -> Data Type Conversion/1
  Constant/1 -> Switch/3
  Sum/1 -> Cumulative Sum/1
  Switch/1 -> Bias/1
  Unit Delay/1 -> Sum/2
  Unit Delay1/1 -> Sum/1
  Constant1/1 -> Sum1/2
  Data Type Conversion/1 -> Sum1/1
  Sum1/1 -> Product/2, Switch/2
  FTExp/1 -> Unit Delay1/1
  FT/1 -> Unit Delay/1

== system wamjc7/Get Arm State/Get FT/Get Force Torque ==
  Enable : EnablePort
  Constant : Constant  Value=256
  Constant1 : Constant  Value=4096
  Constant2 : Constant  Value=rotFT2Hand
  Divide : Product  Inputs=*/
  Divide1 : Product  Inputs=*/
  DocBlock : simulink/Model-Wide Utilities/DocBlock  DocumentType=Text
  Mux : Mux  Inputs=2
  Recieve and Unpack  Forces and Torques : Subsystem
  Rotate To Hand Frame : Product  Multiplication=Matrix(*)
  Rotate To Hand Frame1 : Product  Multiplication=Matrix(*)
  Send Get FT : Subsystem
  FT : Outport
  OriginalFilter : Outport  Port=2
  NewFilter : Outport  Port=3
  wires:
  Constant/1 -> Divide/2
  Constant1/1 -> Divide1/2
  Rotate To Hand Frame/1 -> Mux/1
  Rotate To Hand Frame1/1 -> Mux/2
  Constant2/1 -> Rotate To Hand Frame1/1, Rotate To Hand Frame/1
  Recieve and Unpack  Forces and Torques/2(Tau) -> Divide1/1
  Recieve and Unpack  Forces and Torques/1(F) -> Divide/1
  Divide/1 -> Rotate To Hand Frame/2
  Divide1/1 -> Rotate To Hand Frame1/2
  Mux/1 -> FT/1, OriginalFilter/1, NewFilter/1

== system wamjc7/Get Arm State/Get FT/Tare FT Sensor ==
  Enable : EnablePort
  ANY VALUE : Constant  Value=[0]  OutDataTypeStr=uint8
  Bit Packing : xpcutilitieslib/Bit Packing   MaskBitPatterns={[0:7] [8:39] [40:55]}  MaskPackDataType=double  MaskPackDataSize=[1]
  Data Type Conversion1 : DataTypeConversion  OutMin=[-8191]  OutMax=[8191]  OutDataTypeStr=int32  RndMeth=Zero
  Send To FT : xpclib/CAN/Softing/CAN-AC2-PCI SJA 1000/Send   board=1  canPort=CAN 1  range=Standard (11-bit)  ids=bin2dec('00000001000')  sizes=[8]  output=off  ts=sample_time  ididx=[0]
  TARE FT : Constant  Value=[182]  OutDataTypeStr=uint8
  wires:
  TARE FT/1 -> Bit Packing/1
  Bit Packing/1 -> Send To FT/1
  ANY VALUE/1 -> Data Type Conversion1/1
  Data Type Conversion1/1 -> Bit Packing/2, Bit Packing/3

== system wamjc7/Get Arm State/Get Gripper Status/Send To MATLAB ==
  UDP : Inport
  Trigger : TriggerPort
  Send to MATLAB : xpclib/UDP/Send  ipAddress=192.168.1.11  ipPort=1501  localPort=-1  vblLen=off  sampletime=-1
  wires:
  UDP/1 -> Send to MATLAB/1

== system wamjc7/Get Arm State/Get Gripper Status/Update Force ==
  params : Inport
  Enable : EnablePort
  Data Type Conversion : DataTypeConversion
  Gripper Force : Outport
  wires:
  params/1 -> Data Type Conversion/1
  Data Type Conversion/1 -> Gripper Force/1

== system wamjc7/Get Arm State/Get Gripper Status/Update Position ==
  params : Inport
  Enable : EnablePort
  Constant : Constant  Value=.001
  Data Type Conversion : DataTypeConversion
  Product : Product  RndMeth=Zero
  Position : Outport
  wires:
  params/1 -> Data Type Conversion/1
  Product/1 -> Position/1
  Constant/1 -> Product/2
  Data Type Conversion/1 -> Product/1

== system wamjc7/Get Arm State/Get Joint Positions/Filter Bad Readings ==
  qM_in : Inport
  Abs : Abs
  Compare To Constant : simulink/Logic and Bit Operations/Compare To Constant  relop=<  const=enc_per_rev/4  OutDataTypeStr=uint8
  Subtract : Sum  Inputs=+-
  Switch : Switch  Criteria=u2 ~= 0
  Unit Delay : UnitDelay  SampleTime=-1
  qM_out : Outport
  wires:
  Unit Delay/1 -> Subtract/2, Switch/3
  Subtract/1 -> Abs/1
  Abs/1 -> Compare To Constant/1
  Compare To Constant/1 -> Switch/2
  qM_in/1 -> Unit Delay/1, Subtract/1, Switch/1
  Switch/1 -> qM_out/1

== system wamjc7/Get Arm State/Get Joint Positions/Motor Counts to Joint Radians ==
  qM : Inport
  Add : Sum
  DocBlock : simulink/Model-Wide Utilities/DocBlock  DocumentType=Text
      content=|
      | Here we do the simple conversion from motor position to joint position,
      | then convert encoder counts to joint radians, then account for the offset
      | in the home position to finally output the joint position in radians. The
      | M2J position matrix can be found in the documentation. Joint 4 has a -18 as
      | opposed to +18 because the motor was reversed at one point during a repair.
      | I believe newer models of the WAM adhere to this -18.
  M2J Position Matrix : Constant  Value=arm_m2jp
  Matrix Multiply : Product  Multiplication=Matrix(*)
  Product : Product  OutMin=[-8192]  OutMax=[8191]  RndMeth=Zero
  cts2rad : Constant  Value=2*pi/enc_per_rev
  home : Constant  Value=arm_home
  qJ : Outport
  wires:
  qM/1 -> Product/2
  Add/1 -> qJ/1
  Matrix Multiply/1 -> Add/2
  home/1 -> Add/1
  cts2rad/1 -> Product/1
  M2J Position Matrix/1 -> Matrix Multiply/1
  Product/1 -> Matrix Multiply/2

== system wamjc7/Get Arm State/Get Joint Positions/Recieve and Unpack  Motor Positions ==
  CAN bit-unpacking {1..7} (7 alike) : xpclib/CAN/Utilities/CAN bit-unpacking   bitpatterns={ [16:23, 8:15, 0:5,-1, -1] }  dtypes={ 'int32'}
  Data Type Conversion : DataTypeConversion  OutDataTypeStr=double
  DocBlock : simulink/Model-Wide Utilities/DocBlock  DocumentType=Text
  Mux1 : Mux  Inputs=7
  "Receive position " : xpclib/CAN/Softing/CAN-AC2-PCI SJA 1000/Receive   board=1  canPort=CAN 1  range=Standard (11-bit)  ids=[bin2dec('10000100011'),bin2dec('10001000011'),bin2dec('10001100011'),bin2dec('10010000011'),bin2dec('10010100011'),bin2dec('10011000011'),bin2dec('10011100011')]  lengths=0  output=Data  inten=on  ts=sample_time  ididx=[0,1,2,3,5,6,7]
  qM : Outport
  wires:
  Mux1/1 -> Data Type Conversion/1
  "Receive position "/1 -> CAN bit-unpacking 4/1
  "Receive position "/2 -> CAN bit-unpacking 1/1
  "Receive position "/3 -> CAN bit-unpacking 2/1
  "Receive position "/4 -> CAN bit-unpacking 3/1
  CAN bit-unpacking 4/1 -> Mux1/1
  CAN bit-unpacking 1/1 -> Mux1/2
  CAN bit-unpacking 2/1 -> Mux1/3
  CAN bit-unpacking 3/1 -> Mux1/4
  Data Type Conversion/1 -> qM/1
  "Receive position "/5 -> CAN bit-unpacking 5/1
  "Receive position "/6 -> CAN bit-unpacking 6/1
  "Receive position "/7 -> CAN bit-unpacking 7/1
  CAN bit-unpacking 5/1 -> Mux1/5
  CAN bit-unpacking 6/1 -> Mux1/6
  CAN bit-unpacking 7/1 -> Mux1/7

== system wamjc7/Get Arm State/Get Joint Positions/Send Get Position ==
  Bit Packing : xpcutilitieslib/Bit Packing   MaskBitPatterns={[0:7]}  MaskPackDataType=double  MaskPackDataSize=[1]
  DocBlock : simulink/Model-Wide Utilities/DocBlock  DocumentType=Text
  Send to all motors : xpclib/CAN/Softing/CAN-AC2-PCI SJA 1000/Send   board=1  canPort=CAN 1  range=Standard (11-bit)  ids=1024  sizes=[1]  output=off  ts=sample_time  ididx=[2]
  get position : Constant  Value=[48]  OutDataTypeStr=int8
  wires:
  get position/1 -> Bit Packing/1
  Bit Packing/1 -> Send to all motors/1

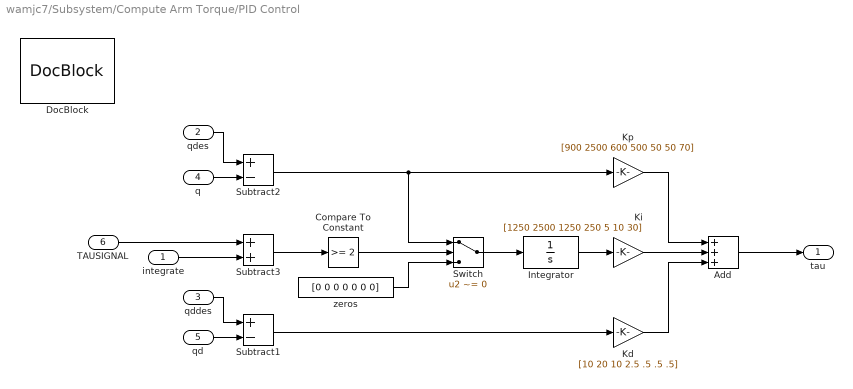
== system wamjc7/Subsystem/Compute Arm Torque/PID Control ==
  integrate : Inport
  qdes : Inport  Port=2
  qddes : Inport  Port=3
  q : Inport  Port=4
  qd : Inport  Port=5
  TAUSIGNAL : Inport  Port=6
  Add : Sum  Inputs=+++
  Compare To Constant : simulink/Logic and Bit Operations/Compare To Constant  relop=>=  const=2  OutDataTypeStr=uint8
  DocBlock : simulink/Model-Wide Utilities/DocBlock  DocumentType=Text
      content=|
      | This is the PID control portion. Desired position comes from the UDP
      | receive block. For now the desired velocity is zero, but eventually we will
      | work in parabolic blending at trajectory points. The integral term is
      | switched off if the WAM is in Shift-Idle mode to avoid integrator windup.
      | There is also a saturation limit on the integration. Finally, the output is
      | the desired joint accelerations which is fed to Recursive Newton Euler.
  Integrator : Integrator  LimitOutput=on  UpperSaturationLimit=0.01  LowerSaturationLimit=-0.01
  Kd : Gain  Gain=[10 20 10 2.5 .5 .5 .5]
  Ki : Gain  Gain=[1250 2500 1250 250 5 10 30]
  Kp : Gain  Gain=[900 2500 600 500 50 50 70]
  Subtract1 : Sum  Inputs=+-
  Subtract2 : Sum  Inputs=+-
  Subtract3 : Sum
  Switch : Switch  Criteria=u2 ~= 0  Threshold=2
  zeros : Constant  Value=[0 0 0 0 0 0 0]  OutDataTypeStr=double
  tau : Outport
  wires:
  Subtract2/1 -> Switch/1, Kp/1
  zeros/1 -> Switch/3
  Add/1 -> tau/1
  qd/1 -> Subtract1/2
  Switch/1 -> Integrator/1
  Kp/1 -> Add/1
  Ki/1 -> Add/2
  Kd/1 -> Add/3
  Subtract1/1 -> Kd/1
  Integrator/1 -> Ki/1
  q/1 -> Subtract2/2
  qdes/1 -> Subtract2/1
  qddes/1 -> Subtract1/1
  Subtract3/1 -> Compare To Constant/1
  Compare To Constant/1 -> Switch/2
  TAUSIGNAL/1 -> Subtract3/1
  integrate/1 -> Subtract3/2

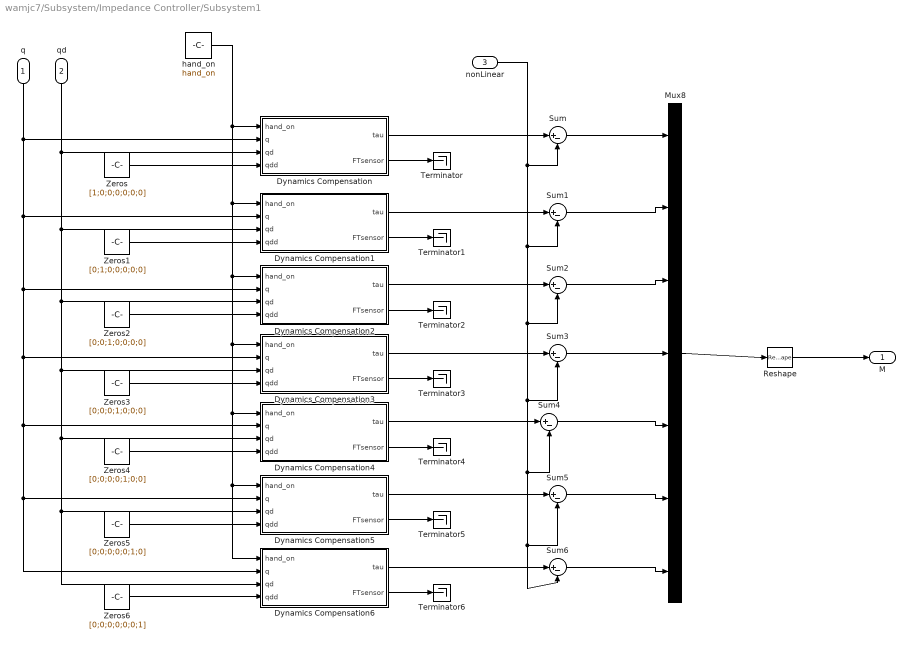
== system wamjc7/Subsystem/Impedance Controller/Subsystem1 ==
  q : Inport
  qd : Inport  Port=2
  nonLinear : Inport  Port=3
  Dynamics Compensation : MATLAB Function  TreatAsAtomicUnit=on
  Dynamics Compensation1 : MATLAB Function  TreatAsAtomicUnit=on
  Dynamics Compensation2 : MATLAB Function  TreatAsAtomicUnit=on
  Dynamics Compensation3 : MATLAB Function  TreatAsAtomicUnit=on
  Dynamics Compensation4 : MATLAB Function  TreatAsAtomicUnit=on
  Dynamics Compensation5 : MATLAB Function  TreatAsAtomicUnit=on
  Dynamics Compensation6 : MATLAB Function  TreatAsAtomicUnit=on
  Mux8 : Mux  Inputs=7
  Reshape : Reshape  OutputDimensionality=Customize  OutputDimensions=[7,7]
  Sum{,1..6} (7 alike) : Sum  Inputs=|+-
  Terminator{,1..6} (7 alike) : Terminator
  Zeros : Constant  Value=[1;0;0;0;0;0;0]
  Zeros1 : Constant  Value=[0;1;0;0;0;0;0]
  Zeros2 : Constant  Value=[0;0;1;0;0;0;0]
  Zeros3 : Constant  Value=[0;0;0;1;0;0;0]
  Zeros4 : Constant  Value=[0;0;0;0;1;0;0]
  Zeros5 : Constant  Value=[0;0;0;0;0;1;0]
  Zeros6 : Constant  Value=[0;0;0;0;0;0;1]
  hand_on : Constant  Value=hand_on
  M : Outport
  wires:
  Reshape/1 -> M/1
  Mux8/1 -> Reshape/1
  Sum5/1 -> Mux8/6
  Sum4/1 -> Mux8/5
  Sum3/1 -> Mux8/4
  Sum2/1 -> Mux8/3
  Sum1/1 -> Mux8/2
  Sum6/1 -> Mux8/7
  Sum/1 -> Mux8/1
  nonLinear/1 -> Sum6/2, Sum5/2, Sum4/2, Sum3/2, Sum2/2, Sum1/2, Sum/2
  Dynamics Compensation6/1(tau) -> Sum6/1
  Dynamics Compensation5/1(tau) -> Sum5/1
  Dynamics Compensation4/1(tau) -> Sum4/1
  Dynamics Compensation3/1(tau) -> Sum3/1
  Dynamics Compensation2/1(tau) -> Sum2/1
  Dynamics Compensation1/1(tau) -> Sum1/1
  Dynamics Compensation/1(tau) -> Sum/1
  qd/1 -> Dynamics Compensation1/3(qd), Dynamics Compensation4/3(qd), Dynamics Compensation5/3(qd), Dynamics Compensation6/3(qd), Dynamics Compensation3/3(qd), Dynamics Compensation2/3(qd), Dynamics Compensation/3(qd)
  q/1 -> Dynamics Compensation4/2(q), Dynamics Compensation5/2(q), Dynamics Compensation6/2(q), Dynamics Compensation3/2(q), Dynamics Compensation2/2(q), Dynamics Compensation1/2(q), Dynamics Compensation/2(q)
  Zeros6/1 -> Dynamics Compensation6/4(qdd)
  Zeros4/1 -> Dynamics Compensation4/4(qdd)
  Zeros3/1 -> Dynamics Compensation3/4(qdd)
  Zeros2/1 -> Dynamics Compensation2/4(qdd)
  Zeros1/1 -> Dynamics Compensation1/4(qdd)
  Zeros/1 -> Dynamics Compensation/4(qdd)
  hand_on/1 -> Dynamics Compensation/1(hand_on), Dynamics Compensation1/1(hand_on), Dynamics Compensation2/1(hand_on), Dynamics Compensation3/1(hand_on), Dynamics Compensation4/1(hand_on), Dynamics Compensation5/1(hand_on), Dynamics Compensation6/1(hand_on)
  Zeros5/1 -> Dynamics Compensation5/4(qdd)
  Dynamics Compensation/2(FTsensor) -> Terminator/1
  Dynamics Compensation1/2(FTsensor) -> Terminator1/1
  Dynamics Compensation2/2(FTsensor) -> Terminator2/1
  Dynamics Compensation3/2(FTsensor) -> Terminator3/1
  Dynamics Compensation4/2(FTsensor) -> Terminator4/1
  Dynamics Compensation5/2(FTsensor) -> Terminator5/1
  Dynamics Compensation6/2(FTsensor) -> Terminator6/1

== system wamjc7/Subsystem/Plan Arm Trajectory/Send Execution Result ==
  Done : Inport
  Execution Status : Inport  Port=2
  Contact : Inport  Port=3
  t : Inport  Port=4
  Detect Change : simulink/Logic and Bit Operations/Detect Change  vinit=0  InputProcessing=Inherited  OutDataTypeStr=uint8
  Determine Execution Result : MATLAB Function  TreatAsAtomicUnit=on
  Enabled Subsystem : Subsystem  TreatAsAtomicUnit=on
  wires:
  Done/1 -> Detect Change/1, Determine Execution Result/1(Done)
  Execution Status/1 -> Determine Execution Result/3(ExecutionStatus)
  Determine Execution Result/2(result) -> Enabled Subsystem/1(ExectuionResult)
  Determine Execution Result/1(sendPacket) -> Enabled Subsystem/Enable
  Detect Change/1 -> Determine Execution Result/2(DoneChanged)
  Contact/1 -> Determine Execution Result/4(contact)
  t/1 -> Determine Execution Result/5(t)
